simulink model "AdmittanceScanPRBS"  (R2025a)
settings: Solver=VariableStepAuto  StartTime=0.0  StopTime=Tsim  RelTol=1e-3
PreLoadFcn:
  | SimulationTime = 10;
  | AdmittanceScanParameters;
undefined symbols (not defined in the file): Array, Base, BatteryInverter, DiscIntNeverNeededParam, ee_sli_rtmsupport, feeder, fRT, frt, gcbh, GFLBatteryController, GFMBatteryController, gGFM, grid, Grid, line, loadpq, loadstep1, loadstep2, lvrt, LVRT, mGFM, Panel, pll, pmsm, PVController, PVInverter, PVTransformer, scan, time, Ts, VSMbase, windController, windTurbine
libraries: ee_lib x19, eeGeneralControl x17, nesl_utility x16, fl_lib x10, eeTransforms x9, simulink x8, slpidlib x2, batteryecm_lib x1, simulink_extras x1, eePowerMeasurement x1
(part 4 of 4)

== system AdmittanceScanPRBS/Renewable Plant/PV Plant/60 MWhr Battery Energy Storage/Variant Subsystem/Grid Forming VSM/GridFormingController/Power Control/ReactiveControl ==
  note: Vs-delV
  Qref : Inport
  Qmeas : Inport  Port=2
  Constant : Constant  Value=voltreference
  Constant2 : Constant  Value=0
  Gain : Gain  Gain=QVoltDroop
  Low-Pass Filter (Discrete or Continuous) : eeGeneralControl/Low-Pass Filter (Discrete or Continuous)  K=1  T=QVoltFilterTC  B=inf  A=-inf  init_option=Specify as parameter  x0=0  Ts=activePowerSampleTime
  Rate Transition : RateTransition
  Rate Transition1 : RateTransition
  Saturation1 : Saturate  UpperLimit=(dcBusVoltage/2)/(sqrt(2/3)*girdLineVoltage)  LowerLimit=-(dcBusVoltage/2)/(sqrt(2/3)*girdLineVoltage)
  Sum : Sum  Inputs=|+-
  Sum1 : Sum  Inputs=|++
  Vmd : Outport
  Vmq : Outport  Port=2
  wires:
  Sum/1 -> Gain/1
  Qmeas/1 -> Low-Pass Filter (Discrete or Continuous)/1
  Low-Pass Filter (Discrete or Continuous)/1 -> Rate Transition1/1
  Gain/1 -> Sum1/1
  Sum1/1 -> Saturation1/1  "Q"
  Constant/1 -> Sum1/2
  Constant2/1 -> Vmq/1
  Qref/1 -> Rate Transition/1
  Saturation1/1 -> Vmd/1
  Rate Transition/1 -> Sum/1
  Rate Transition1/1 -> Sum/2

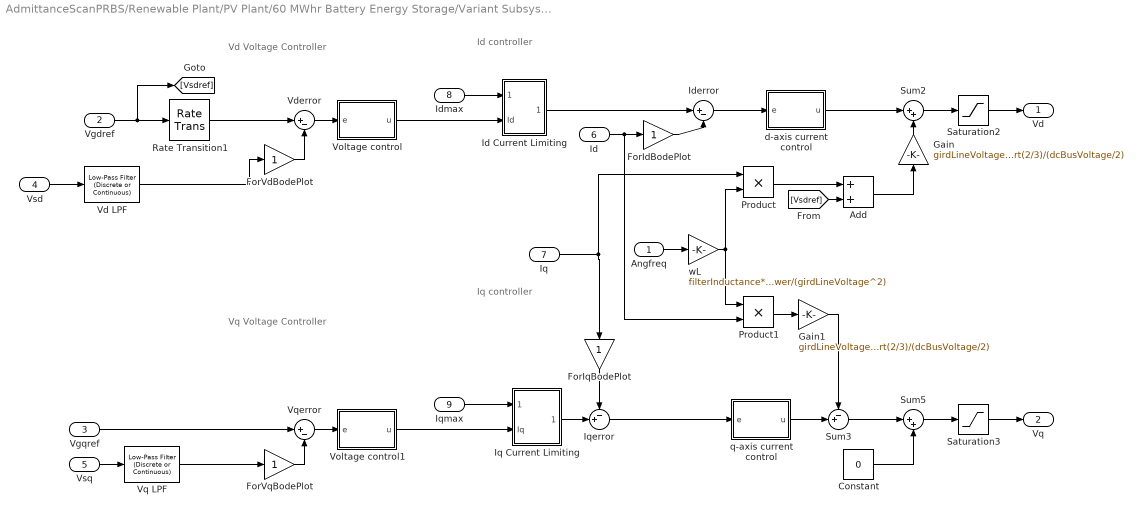
== system AdmittanceScanPRBS/Renewable Plant/PV Plant/60 MWhr Battery Energy Storage/Variant Subsystem/Grid Forming VSM/GridFormingController/VoltageCurrentControl/Controller ==
  note: Id controller
  note: Vd Voltage Controller
  note: Iq controller
  note: Vq Voltage Controller
  Angfreq : Inport
  Vgdref : Inport  Port=2
  Vgqref : Inport  Port=3
  Vsd : Inport  Port=4
  Vsq : Inport  Port=5
  Id : Inport  Port=6
  Iq : Inport  Port=7
  Idmax : Inport  Port=8
  Iqmax : Inport  Port=9
  Add : Sum
  Constant : Constant  Value=0  SampleTime=currentControlTs
  ForIdBodePlot : Gain
  ForIqBodePlot : Gain
  ForVdBodePlot : Gain
  ForVqBodePlot : Gain
  Gain : Gain  Gain=girdLineVoltage*sqrt(2/3)/(dcBusVoltage/2)
  Gain1 : Gain  Gain=girdLineVoltage*sqrt(2/3)/(dcBusVoltage/2)
  Id Current Limiting : Subsystem
  Iderror : Sum  Inputs=|+-
  Iq Current Limiting : Subsystem
  Iqerror : Sum  Inputs=-+|
  Product : Product
  Product1 : Product
  Rate Transition1 : RateTransition
  Saturation2 : Saturate  UpperLimit=4  LowerLimit=-3
  Saturation3 : Saturate  UpperLimit=3  LowerLimit=-3
  Sum2 : Sum  Inputs=|++
  Sum3 : Sum  Inputs=-+|
  Sum5 : Sum  Inputs=|++
  Vd LPF : eeGeneralControl/Low-Pass Filter (Discrete or Continuous)  K=1  T=vdvqLPFTimeConst  B=inf  A=-inf  init_option=Specify as parameter  x0=0  Ts=voltControlTs
  Vderror : Sum  Inputs=|+-
  Voltage control : Subsystem
  Voltage control1 : Subsystem
  Vq LPF : eeGeneralControl/Low-Pass Filter (Discrete or Continuous)  K=1  T=vdvqLPFTimeConst  B=inf  A=-inf  init_option=Inherited from block input  x0=0  Ts=voltControlTs
  Vqerror : Sum  Inputs=|+-
  d-axis current control : Subsystem
  q-axis current control : Subsystem
  wL : Gain  Gain=filterInductance*power/(girdLineVoltage^2)
  Vd : Outport  VectorParamsAs1DForOutWhenUnconnected=off
  Vq : Outport  Port=2  VectorParamsAs1DForOutWhenUnconnected=off
  wires:
  Iqerror/1 -> q-axis current control/1(e)
  wL/1 -> Product1/1, Product/2
  Iq/1 -> ForIqBodePlot/1, Product/1
  Angfreq/1 -> wL/1
  Constant/1 -> Sum5/2
  Iderror/1 -> d-axis current control/1(e)
  Saturation3/1 -> Vq/1
  Saturation2/1 -> Vd/1
  Product1/1 -> Gain1/1
  Product/1 -> Add/1
  d-axis current control/1(u) -> Sum2/1
  Sum2/1 -> Saturation2/1
  q-axis current control/1(u) -> Sum3/2
  Sum3/1 -> Sum5/1
  Sum5/1 -> Saturation3/1
  Vsq/1 -> Vq LPF/1
  Id/1 -> Product1/2, ForIdBodePlot/1
  Vderror/1 -> Voltage control/1(e)
  Iqmax/1 -> Iq Current Limiting/1(Imax)
  Vgqref/1 -> Vqerror/1
  Vqerror/1 -> Voltage control1/1(e)
  Gain1/1 -> Sum3/1
  [Vsdref] -> Add/2
  Add/1 -> Gain/1
  Gain/1 -> Sum2/2
  Voltage control/1(u) -> Id Current Limiting/2(Id)
  Idmax/1 -> Id Current Limiting/1(Imax)
  Iq Current Limiting/1(Iqref) -> Iqerror/2
  Voltage control1/1(u) -> Iq Current Limiting/2(Iq)
  Vsd/1 -> Vd LPF/1
  ForVdBodePlot/1 -> Vderror/2
  ForVqBodePlot/1 -> Vqerror/2
  ForIdBodePlot/1 -> Iderror/2
  ForIqBodePlot/1 -> Iqerror/1
  Id Current Limiting/1(Idref) -> Iderror/1
  Vq LPF/1 -> ForVqBodePlot/1
  Vgdref/1 -> Rate Transition1/1, [Vsdref]
  Vd LPF/1 -> ForVdBodePlot/1
  Rate Transition1/1 -> Vderror/1

== system AdmittanceScanPRBS/Renewable Plant/PV Plant/60 MWhr Battery Energy Storage/Variant Subsystem/Grid Forming VSM/GridFormingController/VoltageCurrentControl/Modulation Signal ==
  Vd : Inport
  Vq : Inport  Port=2
  Angle : Inport  Port=3
  Constant : Constant  Value=0
  Inverse Park Transform : eeTransforms/Inverse Park Transform  AxisAlignment=D-axis  PowerInvariant=off
  Mux1 : Mux  Inputs=3
  Saturation2 : Saturate  UpperLimit=1  LowerLimit=-1
  mabc : Outport  VectorParamsAs1DForOutWhenUnconnected=off
  wires:
  Inverse Park Transform/1 -> Saturation2/1
  Mux1/1 -> Inverse Park Transform/1
  Angle/1 -> Inverse Park Transform/2
  Saturation2/1 -> mabc/1
  Constant/1 -> Mux1/3
  Vd/1 -> Mux1/1
  Vq/1 -> Mux1/2

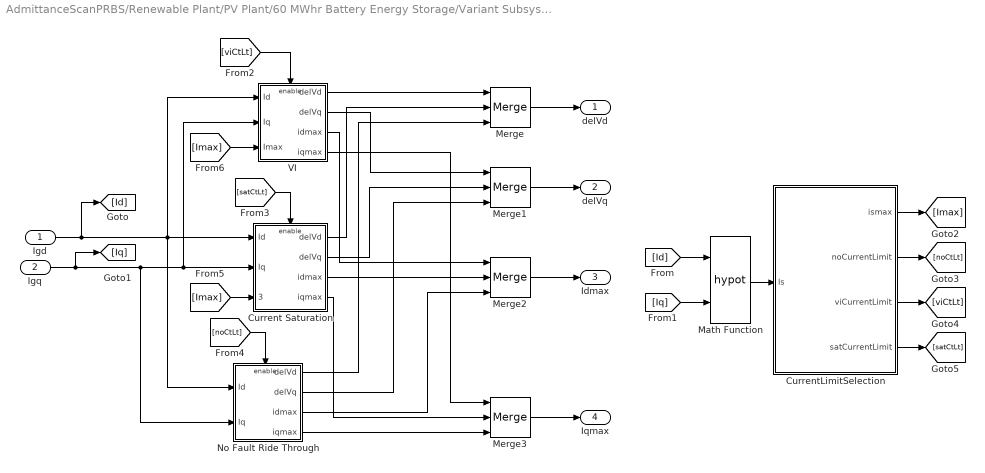
== system AdmittanceScanPRBS/Renewable Plant/PV Plant/60 MWhr Battery Energy Storage/Variant Subsystem/Grid Forming VSM/GridFormingController/Current Limiting/CurrentLimitingMethod/currentLimitAndVirtual ==
  Igd : Inport
  Igq : Inport  Port=2
  Current Saturation : Subsystem
  CurrentLimitSelection : Stateflow chart  TreatAsAtomicUnit=on
  Math Function : Math  Operator=hypot
  Merge{,1..3} (4 alike) : Merge  Inputs=3
  No Fault Ride Through : Subsystem
  VI : Subsystem
  delVd : Outport
  delVq : Outport  Port=2
  Idmax : Outport  Port=3
  Iqmax : Outport  Port=4
  wires:
  Merge2/1 -> Idmax/1
  Igq/1 -> Current Saturation/2(Iq), VI/2(Iq), No Fault Ride Through/2(Iq), [Iq]
  Merge1/1 -> delVq/1
  Igd/1 -> VI/1(Id), Current Saturation/1(Id), No Fault Ride Through/1(Id), [Id]
  No Fault Ride Through/1(delVd) -> Merge/3
  No Fault Ride Through/3(idmax) -> Merge2/3
  VI/1(delVd) -> Merge/1
  [Iq] -> Math Function/2
  [Id] -> Math Function/1
  Current Saturation/1(delVd) -> Merge/2
  Current Saturation/4(iqmax) -> Merge3/2
  Merge/1 -> delVd/1
  VI/2(delVq) -> Merge1/1
  Current Saturation/3(idmax) -> Merge2/2
  VI/4(iqmax) -> Merge3/1
  VI/3(idmax) -> Merge2/1
  No Fault Ride Through/4(iqmax) -> Merge3/3
  Current Saturation/2(delVq) -> Merge1/2
  Merge3/1 -> Iqmax/1
  No Fault Ride Through/2(delVq) -> Merge1/3
  Math Function/1 -> CurrentLimitSelection/1(Is)
  CurrentLimitSelection/1(ismax) -> [Imax]
  CurrentLimitSelection/2(noCurrentLimit) -> [noCtLt]
  CurrentLimitSelection/3(viCurrentLimit) -> [viCtLt]
  CurrentLimitSelection/4(satCurrentLimit) -> [satCtLt]
  [viCtLt] -> VI/Enable
  [satCtLt] -> Current Saturation/Enable
  [noCtLt] -> No Fault Ride Through/Enable
  [Imax] -> Current Saturation/3(Imaxsat)
  [Imax] -> VI/3(Imax)

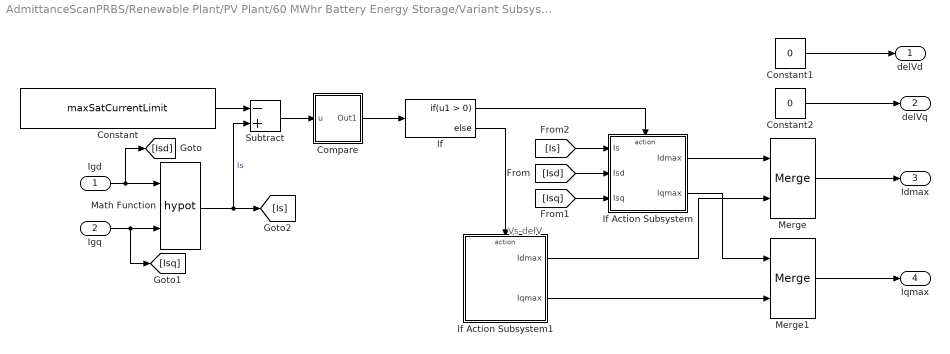
== system AdmittanceScanPRBS/Renewable Plant/PV Plant/60 MWhr Battery Energy Storage/Variant Subsystem/Grid Forming VSM/GridFormingController/Current Limiting/CurrentLimitingMethod/currentSaturation ==
  note: Vs-delV
  Igd : Inport
  Igq : Inport  Port=2
  Compare : Subsystem
  Constant : Constant  Value=maxSatCurrentLimit
  Constant1 : Constant  Value=0
  Constant2 : Constant  Value=0
  If : If
  If Action Subsystem : Subsystem  TreatAsAtomicUnit=on
  If Action Subsystem1 : Subsystem  TreatAsAtomicUnit=on
  Math Function : Math  Operator=hypot
  Merge : Merge
  Merge1 : Merge
  Subtract : Sum  Inputs=-+
  delVd : Outport
  delVq : Outport  Port=2
  Idmax : Outport  Port=3
  Iqmax : Outport  Port=4
  wires:
  Igd/1 -> [Isd], Math Function/1
  Igq/1 -> [Isq], Math Function/2
  Constant/1 -> Subtract/1
  Math Function/1 -> [Is], Subtract/2  "Is"
  If/1 -> If Action Subsystem/Action
  [Isd] -> If Action Subsystem/2(Isd)
  [Isq] -> If Action Subsystem/3(Isq)
  Subtract/1 -> Compare/1(u)
  Compare/1(Out1) -> If/1
  If/2 -> If Action Subsystem1/Action
  [Is] -> If Action Subsystem/1(Is)
  If Action Subsystem/1(Idmax) -> Merge/1
  If Action Subsystem1/1(Idmax) -> Merge/2
  If Action Subsystem/2(Iqmax) -> Merge1/1
  If Action Subsystem1/2(Iqmax) -> Merge1/2
  Constant2/1 -> delVq/1
  Constant1/1 -> delVd/1
  Merge/1 -> Idmax/1
  Merge1/1 -> Iqmax/1

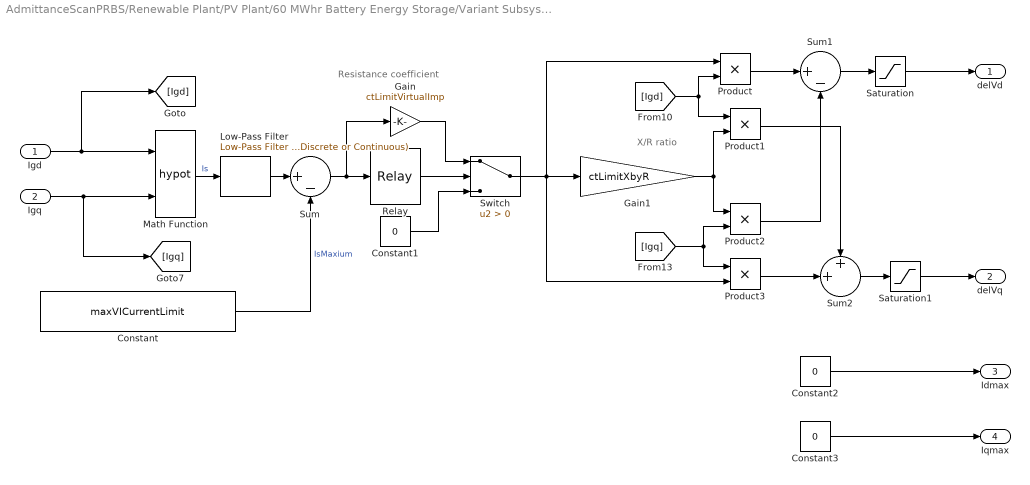
== system AdmittanceScanPRBS/Renewable Plant/PV Plant/60 MWhr Battery Energy Storage/Variant Subsystem/Grid Forming VSM/GridFormingController/Current Limiting/CurrentLimitingMethod/virtualImpedance ==
  note: X/R ratio
  note: Resistance coefficient
  Igd : Inport
  Igq : Inport  Port=2
  Constant : Constant  Value=maxVICurrentLimit
  Constant1 : Constant  Value=0
  Constant2 : Constant  Value=0
  Constant3 : Constant  Value=0
  Gain : Gain  Gain=ctLimitVirtualImp
  Gain1 : Gain  Gain=ctLimitXbyR
  Low-Pass Filter : eeGeneralControl/Low-Pass Filter (Discrete or Continuous)  K=1  T=currentVITimeConst  B=inf  A=-inf  init_option=Inherited from block input  x0=0  Ts=-1
  Math Function : Math  Operator=hypot
  Product{,1..3} (4 alike) : Product
  Relay : Relay  OnSwitchValue=0.01  OffSwitchValue=-0.05
  Saturation : Saturate  UpperLimit=1  LowerLimit=-1
  Saturation1 : Saturate  UpperLimit=1  LowerLimit=-1
  Sum : Sum  Inputs=|+-
  Sum1 : Sum  Inputs=|+-
  Sum2 : Sum  Inputs=++|
  Switch : Switch  Criteria=u2 > Threshold  SaturateOnIntegerOverflow=off  InputSameDT=off
  delVd : Outport
  delVq : Outport  Port=2
  Idmax : Outport  Port=3
  Iqmax : Outport  Port=4
  wires:
  Sum/1 -> Gain/1, Relay/1
  Igq/1 -> [Igq], Math Function/2
  Product1/1 -> Sum2/1
  Gain1/1 -> Product1/2, Product2/1
  Sum1/1 -> Saturation/1
  Product/1 -> Sum1/1
  Product2/1 -> Sum1/2
  Constant/1 -> Sum/2  "IsMaxium"
  Math Function/1 -> Low-Pass Filter/1  "Is"
  [Igq] -> Product3/1, Product2/2
  Switch/1 -> Gain1/1, Product3/2, Product/1
  [Igd] -> Product1/1, Product/2
  Constant2/1 -> Idmax/1
  Constant3/1 -> Iqmax/1
  Gain/1 -> Switch/1
  Constant1/1 -> Switch/3
  Igd/1 -> Math Function/1, [Igd]
  Saturation1/1 -> delVq/1
  Relay/1 -> Switch/2
  Saturation/1 -> delVd/1
  Low-Pass Filter/1 -> Sum/1
  Product3/1 -> Sum2/2
  Sum2/1 -> Saturation1/1

== system AdmittanceScanPRBS/Renewable Plant/PV Plant/60 MWhr Battery Energy Storage/Variant Subsystem/Grid Forming VSM/GridFormingController/Grid Voltage Reactive Power Support/Modifying Active Power Reference/Computing New Active Power Ref ==
  Iq : Inport
  Vd : Inport  Port=2
  Abs : Abs  SaturateOnIntegerOverflow=off
  Constant : Constant  Value=maxVICurrentLimit*0.96
  Constant1 : Constant  Value=0
  Product : Product
  Sqrt : Sqrt
  Square : Math  Operator=square
  Square1 : Math  Operator=square
  Subtract : Sum  Inputs=-+
  Switch : Switch  Criteria=u2 > Threshold  Threshold=1.15  SaturateOnIntegerOverflow=off  InputSameDT=off
  Pref : Outport
  wires:
  Constant/1 -> Square1/1
  Switch/1 -> Product/2
  Square/1 -> Subtract/1
  Square1/1 -> Subtract/2
  Vd/1 -> Product/1
  Sqrt/1 -> Abs/1
  Iq/1 -> Square/1
  Product/1 -> Pref/1
  Subtract/1 -> Switch/2, Sqrt/1
  Constant1/1 -> Switch/3
  Abs/1 -> Switch/1

== system AdmittanceScanPRBS/Renewable Plant/PV Plant/60 MWhr Battery Energy Storage/Variant Subsystem/Grid Forming VSM/GridFormingController/Grid Voltage Reactive Power Support/Modifying Reactive Power Reference/Changing the Power Reference ==
  Vs : Inport
  Vd : Inport  Port=2
  Pref : Inport  Port=3
  Qref : Inport  Port=4
  Enable : EnablePort
  ActivePowerReference : Subsystem
  Constant1 : Constant  Value=voltreference*0.96
  Estimate Id for Given Iq : Subsystem
  EstimateIqForReactivePower : Subsystem
  Max : MinMax  Function=max  Inputs=2
  Rate Transition1 : RateTransition
  ReactivePowerReference : Subsystem
  Prefv : Outport
  Qrefv : Outport  Port=2
  wires:
  EstimateIqForReactivePower/1(Iq) -> Estimate Id for Given Iq/1(Iq), ReactivePowerReference/2(Iq)
  Constant1/1 -> EstimateIqForReactivePower/1(Vmin)
  Vs/1 -> Rate Transition1/1
  Estimate Id for Given Iq/1(Id) -> ActivePowerReference/1(Id)
  Pref/1 -> ActivePowerReference/3(Pref)
  ReactivePowerReference/1(QrefNew) -> Max/1
  Qref/1 -> Max/2
  Vd/1 -> EstimateIqForReactivePower/2(Vd)
  Max/1 -> Qrefv/1
  ActivePowerReference/1(PrefNew) -> Prefv/1
  Rate Transition1/1 -> EstimateIqForReactivePower/3(Vs), ReactivePowerReference/1(Vd), ActivePowerReference/2(Vd)

== system AdmittanceScanPRBS/Renewable Plant/PV Plant/60 MWhr Battery Energy Storage/Variant Subsystem/Grid Forming VSM/GridFormingController/Grid Voltage Reactive Power Support/Modifying Reactive Power Reference/Hysteresis ==
  Vs : Inport
  AND : Logic  IconShape=distinctive  AllPortsSameDT=off  OutDataTypeStr=boolean
  Compare To Constant : simulink/Logic and Bit Operations/Compare To Constant  relop=<  const=0.9  OutDataTypeStr=boolean
  Compare To Constant1 : simulink/Logic and Bit Operations/Compare To Constant  relop=<  const=0.95  OutDataTypeStr=boolean
  D Latch : simulink_extras/Flip Flops/D Latch
  OR : Logic  Operator=OR  IconShape=distinctive  AllPortsSameDT=off  OutDataTypeStr=boolean
  Terminator : Terminator
  LVFlag : Outport
  wires:
  Compare To Constant1/1 -> AND/1
  D Latch/1 -> AND/2
  AND/1 -> OR/1
  OR/1 -> LVFlag/1
  D Latch/2 -> Terminator/1
  Compare To Constant/1 -> D Latch/1, D Latch/2, OR/2
  Vs/1 -> Compare To Constant1/1, Compare To Constant/1

== system AdmittanceScanPRBS/Renewable Plant/PV Plant/60 MWhr Battery Energy Storage/Variant Subsystem/Grid Forming VSM/GridFormingController/Grid Voltage Reactive Power Support/Modifying Reactive Power Reference/Not Altering the Power Reference ==
  Pref : Inport
  Qref : Inport  Port=2
  Enable : EnablePort
  Prefv : Outport
  Qrefv : Outport  Port=2
  wires:
  Pref/1 -> Prefv/1
  Qref/1 -> Qrefv/1

== system AdmittanceScanPRBS/Renewable Plant/PV Plant/60 MWhr Battery Energy Storage/Variant Subsystem/Grid Forming VSM/GridFormingController/Measurement/Frequency Measurement/Frequency Measurement ==
  abc : Inport
  Constant : Constant
  Discrete-Time Integrator : DiscreteIntegrator  SampleTime=sampleTime  LimitOutput=on  ICPrevOutput=DiscIntNeverNeededParam  ICPrevScaledInput=DiscIntNeverNeededParam
  If : If  IfExpression=u1 > 0.9
  If Action Subsystem : Subsystem  TreatAsAtomicUnit=on
  If Action Subsystem1 : Subsystem  TreatAsAtomicUnit=on
  Merge : Merge
  Postive Sequence : Subsystem
  Freq : Outport
  wires:
  If/1 -> If Action Subsystem/Action
  If/2 -> If Action Subsystem1/Action
  Discrete-Time Integrator/1 -> If Action Subsystem/2(Time), If/1
  abc/1 -> Postive Sequence/1(abc)
  Constant/1 -> Discrete-Time Integrator/1
  If Action Subsystem/1(Freq) -> Merge/1
  If Action Subsystem1/1(Out1) -> Merge/2
  Merge/1 -> Freq/1
  Postive Sequence/1(posSeq) -> If Action Subsystem/1(V)

== system AdmittanceScanPRBS/Renewable Plant/PV Plant/60 MWhr Battery Energy Storage/Variant Subsystem/Grid Forming VSM/GridFormingController/Measurement/abc2dq/Supply Current to dq ==
  abc : Inport
  Angle : Inport  Port=2
  Demux : Demux  Outputs=3
  Park Transform : eeTransforms/Park Transform  AxisAlignment=D-axis  PowerInvariant=off
  Terminator : Terminator
  Igd : Outport  VectorParamsAs1DForOutWhenUnconnected=off
  Igq : Outport  Port=2  VectorParamsAs1DForOutWhenUnconnected=off
  wires:
  Demux/3 -> Terminator/1
  Park Transform/1 -> Demux/1
  Demux/2 -> Igq/1
  Demux/1 -> Igd/1
  abc/1 -> Park Transform/1
  Angle/1 -> Park Transform/2

== system AdmittanceScanPRBS/Renewable Plant/PV Plant/60 MWhr Battery Energy Storage/Variant Subsystem/Grid Forming VSM/GridFormingController/Measurement/abc2dq/Supply Voltage  to dq ==
  Angle : Inport
  abc : Inport  Port=2
  Demux : Demux  Outputs=3
  Park Transform : eeTransforms/Park Transform  AxisAlignment=D-axis  PowerInvariant=off
  Terminator : Terminator
  Vgd : Outport  VectorParamsAs1DForOutWhenUnconnected=off
  Vgq : Outport  Port=2  VectorParamsAs1DForOutWhenUnconnected=off
  wires:
  Demux/3 -> Terminator/1
  Park Transform/1 -> Demux/1
  Demux/2 -> Vgq/1
  Demux/1 -> Vgd/1
  abc/1 -> Park Transform/1
  Angle/1 -> Park Transform/2

== system AdmittanceScanPRBS/Renewable Plant/PV Plant/60 MWhr Battery Energy Storage/Variant Subsystem/Grid Forming VSM/GridFormingController/Power Control/ActivePowerControl/droopControl ==
  Pref : Inport
  Pmeas : Inport  Port=2
  fgrid : Inport  Port=3
  Add : Sum  Inputs=+-
  Constant : Constant
  Constant5 : Constant  Value=pi/2
  Gain : Gain  Gain=powerFreq*2*pi
  Integrator with Wrapped State (Discrete or Continuous) : eeGeneralControl/Integrator with Wrapped State (Discrete or Continuous)  LabelModeActiveChoice=Discrete  WrappedStateUpperValue=2*pi  WrappedStateLowerValue=0  x0=0  Ts=activePowerSampleTime
      settings: LibrarySourceBlock=|
      | ee_sl_lib/General Control/Integrator with
      | Wrapped State
      | (Discrete or Continuous)
  Lead-Lag (Discrete or Continuous) : eeGeneralControl/Lead-Lag (Discrete or Continuous)  T1=droopT1  T2=droopT2  B=inf  A=-inf  init_option=Inherited from block input  x0=0  Ts=activePowerSampleTime
      settings: LibrarySourceBlock=|
      | ee_sl_lib/General Control/Lead-Lag
      | (Discrete or Continuous)
  Low-Pass Filter (Discrete or Continuous) : eeGeneralControl/Low-Pass Filter (Discrete or Continuous)  K=1  T=droopTC  B=inf  A=-inf  init_option=Specify as parameter  x0=0  Ts=activePowerSampleTime
  Sum : Sum  Inputs=|-+
  Sum1 : Sum  Inputs=|-+
  Terminator : Terminator
  mp : Gain  Gain=droopSlope
  Theta : Outport
  w : Outport  Port=2
  wires:
  Low-Pass Filter (Discrete or Continuous)/1 -> Sum1/1
  mp/1 -> Low-Pass Filter (Discrete or Continuous)/1
  Sum/1 -> mp/1
  Pmeas/1 -> Lead-Lag (Discrete or Continuous)/1
  Add/1 -> Theta/1
  Constant5/1 -> Add/2
  Pref/1 -> Sum/1
  Gain/1 -> Integrator with Wrapped State (Discrete or Continuous)/1, w/1
  Lead-Lag (Discrete or Continuous)/1 -> Sum/2
  Integrator with Wrapped State (Discrete or Continuous)/1 -> Add/1
  Constant/1 -> Sum1/2
  Sum1/1 -> Gain/1
  fgrid/1 -> Terminator/1

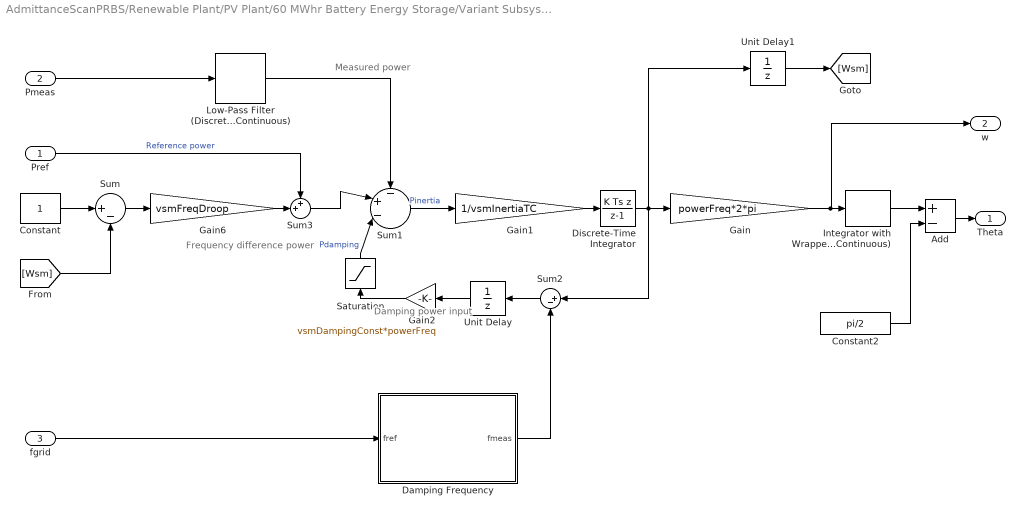
== system AdmittanceScanPRBS/Renewable Plant/PV Plant/60 MWhr Battery Energy Storage/Variant Subsystem/Grid Forming VSM/GridFormingController/Power Control/ActivePowerControl/vsmControl ==
  note: Measured power
  note: Frequency difference power
  note: Damping power input
  Pref : Inport
  Pmeas : Inport  Port=2
  fgrid : Inport  Port=3
  Add : Sum  Inputs=+-
  Constant : Constant
  Constant2 : Constant  Value=pi/2
  Damping Frequency : Subsystem  Variant=on  VariantControlMode=label  VariantControl=Choice  LabelModeActiveChoice=freqMeas
  Discrete-Time Integrator : DiscreteIntegrator  IntegratorMethod=Integration: Backward Euler  InitialCondition=1  SampleTime=activePowerSampleTime  LimitOutput=on  UpperSaturationLimit=1.1  LowerSaturationLimit=0.9  ICPrevOutput=DiscIntNeverNeededParam  ICPrevScaledInput=DiscIntNeverNeededParam
  Gain : Gain  Gain=powerFreq*2*pi
  Gain1 : Gain  Gain=1/vsmInertiaTC
  Gain2 : Gain  Gain=vsmDampingConst*powerFreq
  Gain6 : Gain  Gain=vsmFreqDroop
  Integrator with Wrapped State (Discrete or Continuous) : eeGeneralControl/Integrator with Wrapped State (Discrete or Continuous)  LabelModeActiveChoice=Discrete  WrappedStateUpperValue=2*pi  WrappedStateLowerValue=0  x0=0  Ts=activePowerSampleTime
      settings: LibrarySourceBlock=|
      | ee_sl_lib/General Control/Integrator with
      | Wrapped State
      | (Discrete or Continuous)
  Low-Pass Filter (Discrete or Continuous) : eeGeneralControl/Low-Pass Filter (Discrete or Continuous)  K=1  T=vsmPmeasFilterTC  B=inf  A=-inf  init_option=Specify as parameter  x0=0  Ts=activePowerSampleTime
  Saturation : Saturate  UpperLimit=dampingPowerMaxLimit  LowerLimit=dampingPowerMinLimit
  Sum : Sum  Inputs=|+-
  Sum1 : Sum  Inputs=-+-|
  Sum2 : Sum  Inputs=|+-
  Sum3 : Sum  Inputs=++|
  Unit Delay : UnitDelay  SampleTime=-1  HasFrameUpgradeWarning=on
  Unit Delay1 : UnitDelay  SampleTime=-1  HasFrameUpgradeWarning=on
  Theta : Outport
  w : Outport  Port=2
  wires:
  Integrator with Wrapped State (Discrete or Continuous)/1 -> Add/1
  Sum1/1 -> Gain1/1  "Pinertia"
  Sum/1 -> Gain6/1
  Constant2/1 -> Add/2
  Add/1 -> Theta/1
  Pmeas/1 -> Low-Pass Filter (Discrete or Continuous)/1
  Discrete-Time Integrator/1 -> Gain/1, Unit Delay1/1, Sum2/1
  [Wsm] -> Sum/2
  Low-Pass Filter (Discrete or Continuous)/1 -> Sum1/1
  Pref/1 -> Sum3/1  "Reference power"
  Gain2/1 -> Saturation/1
  Sum3/1 -> Sum1/2
  Sum2/1 -> Unit Delay/1
  Gain1/1 -> Discrete-Time Integrator/1
  Gain/1 -> Integrator with Wrapped State (Discrete or Continuous)/1, w/1
  Unit Delay/1 -> Gain2/1
  Constant/1 -> Sum/1
  Unit Delay1/1 -> [Wsm]
  Saturation/1 -> Sum1/3  "Pdamping"
  Gain6/1 -> Sum3/2
  fgrid/1 -> Damping Frequency/1(fref)
  Damping Frequency/1(fmeas) -> Sum2/2

== system AdmittanceScanPRBS/Renewable Plant/PV Plant/60 MWhr Battery Energy Storage/Variant Subsystem/Grid Forming VSM/GridFormingController/VoltageCurrentControl/Controller/Id Current Limiting ==
  Imax : Inport
  Id : Inport  Port=2
  Abs : Abs  SaturateOnIntegerOverflow=off
  Rate Transition : RateTransition
  Switch : Switch  Criteria=u2 > Threshold  SaturateOnIntegerOverflow=off  InputSameDT=off
  Idref : Outport
  wires:
  Id/1 -> Rate Transition/1
  Abs/1 -> Switch/2
  Imax/1 -> Abs/1, Switch/1
  Switch/1 -> Idref/1
  Rate Transition/1 -> Switch/3

== system AdmittanceScanPRBS/Renewable Plant/PV Plant/60 MWhr Battery Energy Storage/Variant Subsystem/Grid Forming VSM/GridFormingController/VoltageCurrentControl/Controller/Iq Current Limiting ==
  Imax : Inport
  Iq : Inport  Port=2
  Abs : Abs  SaturateOnIntegerOverflow=off
  Switch : Switch  Criteria=u2 > Threshold  SaturateOnIntegerOverflow=off  InputSameDT=off
  Iqref : Outport
  wires:
  Iq/1 -> Switch/3
  Abs/1 -> Switch/2
  Imax/1 -> Abs/1, Switch/1
  Switch/1 -> Iqref/1

== system AdmittanceScanPRBS/Renewable Plant/PV Plant/60 MWhr Battery Energy Storage/Variant Subsystem/Grid Forming VSM/GridFormingController/VoltageCurrentControl/Controller/Voltage control ==
  e : Inport
  Discrete-Time Integrator : DiscreteIntegrator  IntegratorMethod=Integration: Backward Euler  SampleTime=voltControlTs  LimitOutput=on  UpperSaturationLimit=VdMaxCt  LowerSaturationLimit=VdMinCt  ICPrevOutput=DiscIntNeverNeededParam  ICPrevScaledInput=DiscIntNeverNeededParam
  Ki : Gain  Gain=VdIGain
  Kp : Gain  Gain=vdPGain
  Limit : Saturate  UpperLimit=VdMaxCt  LowerLimit=VdMinCt
  Sum7 : Sum  Inputs=|++
  u : Outport  VectorParamsAs1DForOutWhenUnconnected=off
  wires:
  Discrete-Time Integrator/1 -> Sum7/2
  Kp/1 -> Sum7/1
  Limit/1 -> u/1
  Ki/1 -> Discrete-Time Integrator/1
  Sum7/1 -> Limit/1
  e/1 -> Kp/1, Ki/1

== system AdmittanceScanPRBS/Renewable Plant/PV Plant/60 MWhr Battery Energy Storage/Variant Subsystem/Grid Forming VSM/GridFormingController/VoltageCurrentControl/Controller/Voltage control1 ==
  e : Inport
  Discrete-Time Integrator : DiscreteIntegrator  IntegratorMethod=Integration: Backward Euler  SampleTime=voltControlTs  LimitOutput=on  UpperSaturationLimit=VqMaxCt  LowerSaturationLimit=VqMinCt  ICPrevOutput=DiscIntNeverNeededParam  ICPrevScaledInput=DiscIntNeverNeededParam
  Ki : Gain  Gain=VqIGain
  Kp : Gain  Gain=VqPGain
  Limit : Saturate  UpperLimit=VqMaxCt  LowerLimit=VqMinCt
  Sum7 : Sum  Inputs=|++
  u : Outport  VectorParamsAs1DForOutWhenUnconnected=off
  wires:
  Discrete-Time Integrator/1 -> Sum7/2
  Sum7/1 -> Limit/1
  e/1 -> Ki/1, Kp/1
  Kp/1 -> Sum7/1
  Ki/1 -> Discrete-Time Integrator/1
  Limit/1 -> u/1

== system AdmittanceScanPRBS/Renewable Plant/PV Plant/60 MWhr Battery Energy Storage/Variant Subsystem/Grid Forming VSM/GridFormingController/VoltageCurrentControl/Controller/d-axis current control ==
  e : Inport
  Discrete-Time Integrator : DiscreteIntegrator  IntegratorMethod=Integration: Backward Euler  SampleTime=currentControlTs  LimitOutput=on  UpperSaturationLimit=4  LowerSaturationLimit=-4  ICPrevOutput=DiscIntNeverNeededParam  ICPrevScaledInput=DiscIntNeverNeededParam
  Ki : Gain  Gain=IdIGain
  Kp : Gain  Gain=IdPGain
  Limit : Saturate  UpperLimit=4  LowerLimit=-4
  Sum7 : Sum  Inputs=|++
  u : Outport  VectorParamsAs1DForOutWhenUnconnected=off
  wires:
  Discrete-Time Integrator/1 -> Sum7/2
  Sum7/1 -> Limit/1
  e/1 -> Ki/1, Kp/1
  Kp/1 -> Sum7/1
  Limit/1 -> u/1
  Ki/1 -> Discrete-Time Integrator/1

== system AdmittanceScanPRBS/Renewable Plant/PV Plant/60 MWhr Battery Energy Storage/Variant Subsystem/Grid Forming VSM/GridFormingController/VoltageCurrentControl/Controller/q-axis current control ==
  e : Inport
  Discrete-Time Integrator : DiscreteIntegrator  IntegratorMethod=Integration: Backward Euler  SampleTime=currentControlTs  LimitOutput=on  UpperSaturationLimit=3  LowerSaturationLimit=-3  ICPrevOutput=DiscIntNeverNeededParam  ICPrevScaledInput=DiscIntNeverNeededParam
  Ki : Gain  Gain=IqIGain
  Kp : Gain  Gain=IqPGain
  Limit : Saturate  UpperLimit=3  LowerLimit=-3
  Sum7 : Sum  Inputs=|++
  u : Outport  VectorParamsAs1DForOutWhenUnconnected=off
  wires:
  Ki/1 -> Discrete-Time Integrator/1
  Kp/1 -> Sum7/1
  e/1 -> Kp/1, Ki/1
  Sum7/1 -> Limit/1
  Limit/1 -> u/1
  Discrete-Time Integrator/1 -> Sum7/2

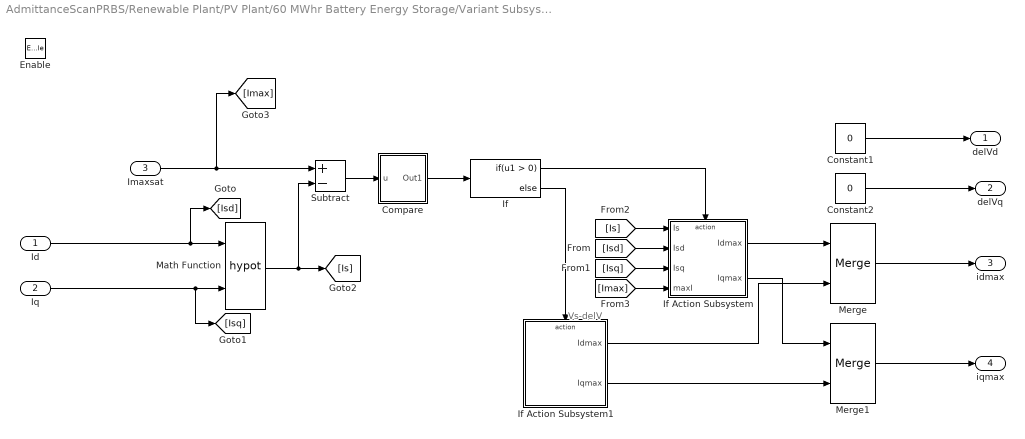
== system AdmittanceScanPRBS/Renewable Plant/PV Plant/60 MWhr Battery Energy Storage/Variant Subsystem/Grid Forming VSM/GridFormingController/Current Limiting/CurrentLimitingMethod/currentLimitAndVirtual/Current Saturation ==
  note: Vs-delV
  Id : Inport
  Iq : Inport  Port=2
  Imaxsat : Inport  Port=3
  Enable : EnablePort
  Compare : Subsystem
  Constant1 : Constant  Value=0
  Constant2 : Constant  Value=0
  If : If
  If Action Subsystem : Subsystem  TreatAsAtomicUnit=on
  If Action Subsystem1 : Subsystem  TreatAsAtomicUnit=on
  Math Function : Math  Operator=hypot
  Merge : Merge
  Merge1 : Merge
  Subtract : Sum  Inputs=+-
  delVd : Outport
  delVq : Outport  Port=2
  idmax : Outport  Port=3
  iqmax : Outport  Port=4
  wires:
  Iq/1 -> [Isq], Math Function/2
  If/1 -> If Action Subsystem/Action
  If Action Subsystem1/1(Idmax) -> Merge/2
  Constant2/1 -> delVq/1
  Math Function/1 -> [Is], Subtract/2
  If/2 -> If Action Subsystem1/Action
  If Action Subsystem/2(Iqmax) -> Merge1/1
  Subtract/1 -> Compare/1(u)
  Compare/1(Out1) -> If/1
  If Action Subsystem/1(Idmax) -> Merge/1
  [Is] -> If Action Subsystem/1(Is)
  Id/1 -> [Isd], Math Function/1
  If Action Subsystem1/2(Iqmax) -> Merge1/2
  Merge/1 -> idmax/1
  [Isd] -> If Action Subsystem/2(Isd)
  Constant1/1 -> delVd/1
  [Isq] -> If Action Subsystem/3(Isq)
  Merge1/1 -> iqmax/1
  Imaxsat/1 -> [Imax], Subtract/1
  [Imax] -> If Action Subsystem/4(maxI)

== system AdmittanceScanPRBS/Renewable Plant/PV Plant/60 MWhr Battery Energy Storage/Variant Subsystem/Grid Forming VSM/GridFormingController/Current Limiting/CurrentLimitingMethod/currentLimitAndVirtual/No Fault Ride Through ==
  Id : Inport
  Iq : Inport  Port=2
  Enable : EnablePort
  Constant{1..4} (4 alike) : Constant  Value=0
  Terminator : Terminator
  Terminator1 : Terminator
  delVd : Outport
  delVq : Outport  Port=2
  idmax : Outport  Port=3
  iqmax : Outport  Port=4
  wires:
  Constant3/1 -> iqmax/1
  Constant2/1 -> idmax/1
  Constant1/1 -> delVd/1
  Constant4/1 -> delVq/1
  Id/1 -> Terminator/1
  Iq/1 -> Terminator1/1

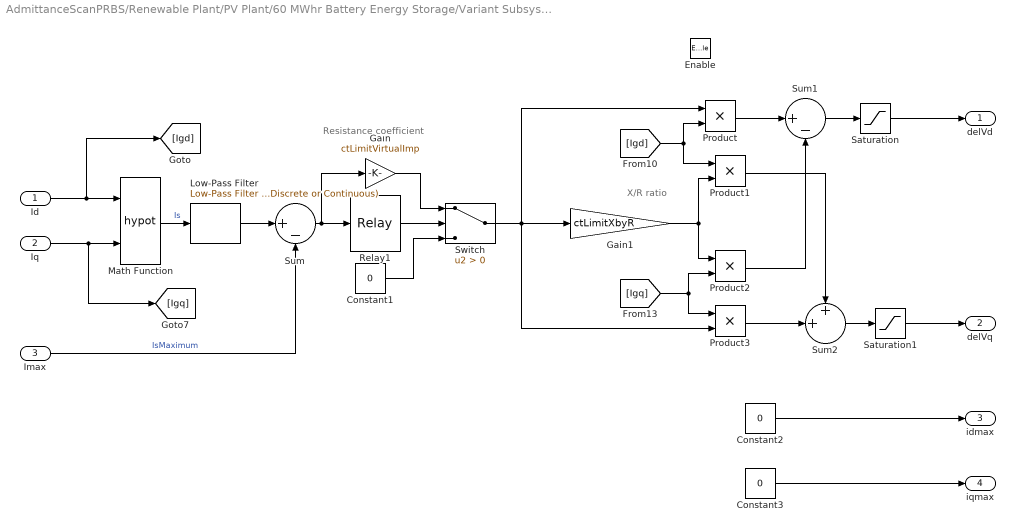
== system AdmittanceScanPRBS/Renewable Plant/PV Plant/60 MWhr Battery Energy Storage/Variant Subsystem/Grid Forming VSM/GridFormingController/Current Limiting/CurrentLimitingMethod/currentLimitAndVirtual/VI ==
  note: Resistance coefficient
  note: X/R ratio
  Id : Inport
  Iq : Inport  Port=2
  Imax : Inport  Port=3
  Enable : EnablePort
  Constant1 : Constant  Value=0
  Constant2 : Constant  Value=0
  Constant3 : Constant  Value=0
  Gain : Gain  Gain=ctLimitVirtualImp
  Gain1 : Gain  Gain=ctLimitXbyR
  Low-Pass Filter : eeGeneralControl/Low-Pass Filter (Discrete or Continuous)  K=1  T=currentVITimeConst  B=inf  A=-inf  init_option=Inherited from block input  x0=0  Ts=-1
  Math Function : Math  Operator=hypot
  Product{,1..3} (4 alike) : Product
  Relay1 : Relay  OnSwitchValue=0.01  OffSwitchValue=-0.1
  Saturation : Saturate  UpperLimit=1  LowerLimit=-1
  Saturation1 : Saturate  UpperLimit=1  LowerLimit=-1
  Sum : Sum  Inputs=|+-
  Sum1 : Sum  Inputs=|+-
  Sum2 : Sum  Inputs=++|
  Switch : Switch  Criteria=u2 > Threshold  SaturateOnIntegerOverflow=off  InputSameDT=off
  delVd : Outport
  delVq : Outport  Port=2
  idmax : Outport  Port=3
  iqmax : Outport  Port=4
  wires:
  Gain1/1 -> Product1/2, Product2/1
  Product3/1 -> Sum2/2
  Id/1 -> Math Function/1, [Igd]
  Sum2/1 -> Saturation1/1
  Sum/1 -> Gain/1, Relay1/1
  Sum1/1 -> Saturation/1
  Product/1 -> Sum1/1
  [Igq] -> Product3/1, Product2/2
  Iq/1 -> [Igq], Math Function/2
  Math Function/1 -> Low-Pass Filter/1  "Is"
  Switch/1 -> Product3/2, Product/1, Gain1/1
  [Igd] -> Product1/1, Product/2
  Saturation1/1 -> delVq/1
  Product1/1 -> Sum2/1
  Product2/1 -> Sum1/2
  Gain/1 -> Switch/1
  Constant1/1 -> Switch/3
  Saturation/1 -> delVd/1
  Constant3/1 -> iqmax/1
  Constant2/1 -> idmax/1
  Relay1/1 -> Switch/2
  Low-Pass Filter/1 -> Sum/1
  Imax/1 -> Sum/2  "IsMaximum"

== system AdmittanceScanPRBS/Renewable Plant/PV Plant/60 MWhr Battery Energy Storage/Variant Subsystem/Grid Forming VSM/GridFormingController/Current Limiting/CurrentLimitingMethod/currentSaturation/Compare ==
  u : Inport
  AND : Logic  IconShape=distinctive  AllPortsSameDT=off  OutDataTypeStr=boolean
  Compare To Constant : simulink/Logic and Bit Operations/Compare To Constant  relop=>  const=ctLimitDelayTime  OutDataTypeStr=boolean
  Data Type Conversion : DataTypeConversion  SaturateOnIntegerOverflow=off  RndMeth=Floor
  Data Type Conversion1 : DataTypeConversion  SaturateOnIntegerOverflow=off  RndMeth=Floor
  Discrete-Time Integrator : DiscreteIntegrator  IntegratorMethod=Integration: Backward Euler  ExternalReset=falling  SampleTime=currentControlTs  LimitOutput=on  UpperSaturationLimit=ctLimitDelayTime*2  LowerSaturationLimit=0  ICPrevOutput=DiscIntNeverNeededParam  ICPrevScaledInput=DiscIntNeverNeededParam
  Relay : Relay  OnSwitchValue=0.005*maxSatCurrentLimit  OffSwitchValue=-1*0.02*maxSatCurrentLimit
  Out1 : Outport
  wires:
  AND/1 -> Data Type Conversion/1
  Relay/1 -> Data Type Conversion1/1
  u/1 -> Relay/1
  Discrete-Time Integrator/1 -> Compare To Constant/1
  Data Type Conversion/1 -> Out1/1
  Data Type Conversion1/1 -> Discrete-Time Integrator/1, AND/1, Discrete-Time Integrator/2
  Compare To Constant/1 -> AND/2

== system AdmittanceScanPRBS/Renewable Plant/PV Plant/60 MWhr Battery Energy Storage/Variant Subsystem/Grid Forming VSM/GridFormingController/Current Limiting/CurrentLimitingMethod/currentSaturation/If Action Subsystem ==
  Is : Inport
  Isd : Inport  Port=2
  Isq : Inport  Port=3
  Action Port : ActionPort
  Constant : Constant  Value=maxSatCurrentLimit
  Divide : Product  Inputs=*/
  Product : Product
  Product1 : Product
  Idmax : Outport
  Iqmax : Outport  Port=2
  wires:
  Constant/1 -> Divide/1
  Is/1 -> Divide/2
  Divide/1 -> Product1/2, Product/1
  Isd/1 -> Product1/1
  Isq/1 -> Product/2
  Product1/1 -> Idmax/1
  Product/1 -> Iqmax/1

== system AdmittanceScanPRBS/Renewable Plant/PV Plant/60 MWhr Battery Energy Storage/Variant Subsystem/Grid Forming VSM/GridFormingController/Current Limiting/CurrentLimitingMethod/currentSaturation/If Action Subsystem1 ==
  Action Port : ActionPort
  Constant3 : Constant  Value=0
  Constant4 : Constant  Value=0
  Idmax : Outport
  Iqmax : Outport  Port=2
  wires:
  Constant4/1 -> Iqmax/1
  Constant3/1 -> Idmax/1

== system AdmittanceScanPRBS/Renewable Plant/PV Plant/60 MWhr Battery Energy Storage/Variant Subsystem/Grid Forming VSM/GridFormingController/Grid Voltage Reactive Power Support/Modifying Reactive Power Reference/Changing the Power Reference/ActivePowerReference ==
  note: Ensure Pref sign is maintained
  Id : Inport
  Vd : Inport  Port=2
  Pref : Inport  Port=3
  Abs1 : Abs  SaturateOnIntegerOverflow=off
  Abs2 : Abs  SaturateOnIntegerOverflow=off
  Min : MinMax  Inputs=2
  Product : Product
  Product2 : Product
  Saturation : Saturate  UpperLimit=1  LowerLimit=-1
  Sign : Signum
  PrefNew : Outport
  wires:
  Pref/1 -> Abs1/1, Sign/1
  Id/1 -> Product/1
  Sign/1 -> Product2/2
  Abs1/1 -> Min/2
  Product/1 -> Abs2/1
  Min/1 -> Product2/1
  Product2/1 -> Saturation/1
  Abs2/1 -> Min/1
  Vd/1 -> Product/2
  Saturation/1 -> PrefNew/1

== system AdmittanceScanPRBS/Renewable Plant/PV Plant/60 MWhr Battery Energy Storage/Variant Subsystem/Grid Forming VSM/GridFormingController/Grid Voltage Reactive Power Support/Modifying Reactive Power Reference/Changing the Power Reference/Estimate Id for Given Iq ==
  Iq : Inport
  Add Constant1 : Bias  Bias=1  SaturateOnIntegerOverflow=off
  Gain : Gain  Gain=-1
  Gain3 : Gain  Gain=0.9
  Sqrt : Sqrt
  Square : Math  Operator=square
  Id : Outport
  wires:
  Square/1 -> Gain/1
  Gain3/1 -> Id/1
  Gain/1 -> Add Constant1/1
  Sqrt/1 -> Gain3/1
  Add Constant1/1 -> Sqrt/1
  Iq/1 -> Square/1

== system AdmittanceScanPRBS/Renewable Plant/PV Plant/60 MWhr Battery Energy Storage/Variant Subsystem/Grid Forming VSM/GridFormingController/Grid Voltage Reactive Power Support/Modifying Reactive Power Reference/Changing the Power Reference/EstimateIqForReactivePower ==
  note: Computing minimum reactive current as per GC0137
  Vmin : Inport
  Vd : Inport  Port=2
  Vs : Inport  Port=3
  Abs : Abs  SaturateOnIntegerOverflow=off
  Add : Sum
  Add Constant : Bias  Bias=1  SaturateOnIntegerOverflow=off
  GC0137 line slope : Gain  Gain=-1.4578
  Low Voltage Support : Subsystem
  Saturation : Saturate  UpperLimit=1  LowerLimit=0
  Iq : Outport
  wires:
  Abs/1 -> GC0137 line slope/1
  GC0137 line slope/1 -> Add Constant/1
  Vs/1 -> Abs/1
  Add/1 -> Saturation/1
  Saturation/1 -> Iq/1
  Add Constant/1 -> Add/2
  Vmin/1 -> Low Voltage Support/1(Vin)
  Vd/1 -> Low Voltage Support/2(Vd)
  Low Voltage Support/1(Iqsupport) -> Add/1

== system AdmittanceScanPRBS/Renewable Plant/PV Plant/60 MWhr Battery Energy Storage/Variant Subsystem/Grid Forming VSM/GridFormingController/Grid Voltage Reactive Power Support/Modifying Reactive Power Reference/Changing the Power Reference/ReactivePowerReference ==
  Vd : Inport
  Iq : Inport  Port=2
  Compute Power : Product
  Constant : Constant  Value=0.3
  Gain2 : Gain  Gain=1.05
  Switch : Switch  Criteria=u2 > Threshold  Threshold=0.3  SaturateOnIntegerOverflow=off  InputSameDT=off
  QrefNew : Outport
  wires:
  Compute Power/1 -> QrefNew/1
  Gain2/1 -> Compute Power/2
  Constant/1 -> Switch/3
  Iq/1 -> Gain2/1
  Vd/1 -> Switch/2, Switch/1
  Switch/1 -> Compute Power/1

== system AdmittanceScanPRBS/Renewable Plant/PV Plant/60 MWhr Battery Energy Storage/Variant Subsystem/Grid Forming VSM/GridFormingController/Measurement/Frequency Measurement/Frequency Measurement/If Action Subsystem ==
  V : Inport
  Time : Inport  Port=2
  Action Port : ActionPort  ActionPortLabel=if(u1 > 0.9)
  Constant1 : Constant  Value=initialFrequency
  Delay : Delay  DelayLength=1
  Delay1 : Delay  DelayLength=1
  Frequency estimation : Subsystem  TreatAsAtomicUnit=on
  Hit Crossing : HitCross
  Switch : Switch  Criteria=u2 > Threshold  Threshold=1  SaturateOnIntegerOverflow=off  InputSameDT=off
  Freq : Outport
  wires:
  V/1 -> Delay/1, Frequency estimation/1(sk), Hit Crossing/1
  Delay1/1 -> Frequency estimation/4(k-1)
  Hit Crossing/1 -> Frequency estimation/Trigger
  Delay/1 -> Frequency estimation/2(sk-1)
  Time/1 -> Switch/2, Delay1/1, Frequency estimation/3(k)
  Frequency estimation/1(f) -> Switch/1
  Constant1/1 -> Switch/3
  Switch/1 -> Freq/1

== system AdmittanceScanPRBS/Renewable Plant/PV Plant/60 MWhr Battery Energy Storage/Variant Subsystem/Grid Forming VSM/GridFormingController/Measurement/Frequency Measurement/Frequency Measurement/If Action Subsystem1 ==
  Action Port : ActionPort  ActionPortLabel=else
  Constant1 : Constant  Value=initialFrequency
  Out1 : Outport
  wires:
  Constant1/1 -> Out1/1

== system AdmittanceScanPRBS/Renewable Plant/PV Plant/60 MWhr Battery Energy Storage/Variant Subsystem/Grid Forming VSM/GridFormingController/Measurement/Frequency Measurement/Frequency Measurement/Postive Sequence ==
  abc : Inport
  Complex to Real-Imag : ComplexToRealImag
  Demux : Demux  Outputs=3
  Symmetrical-Components Transform : eeTransforms/Symmetrical-Components Transform  PowerInvariant=off
      settings: LibrarySourceBlock=|
      | ee_sl_lib/Mathematical
      | Transforms/Symmetrical-Components
      | Transform
  Terminator : Terminator
  Terminator1 : Terminator
  Terminator2 : Terminator
  Transpose : Math  Operator=transpose
  posSeq : Outport
  wires:
  Transpose/1 -> Symmetrical-Components Transform/1
  Symmetrical-Components Transform/1 -> Demux/1
  Complex to Real-Imag/1 -> posSeq/1
  Demux/1 -> Complex to Real-Imag/1
  abc/1 -> Transpose/1
  Complex to Real-Imag/2 -> Terminator/1
  Demux/2 -> Terminator1/1
  Demux/3 -> Terminator2/1

== system AdmittanceScanPRBS/Renewable Plant/PV Plant/60 MWhr Battery Energy Storage/Variant Subsystem/Grid Forming VSM/GridFormingController/Power Control/ActivePowerControl/vsmControl/Damping Frequency ==
  fref : Inport
  ConstantFreqReference : Subsystem  VariantControl=constFreq
  WithFrequencyMeasurement : Subsystem  VariantControl=freqMeas
  fmeas : Outport

== system AdmittanceScanPRBS/Renewable Plant/PV Plant/60 MWhr Battery Energy Storage/Variant Subsystem/Grid Forming VSM/GridFormingController/Current Limiting/CurrentLimitingMethod/currentLimitAndVirtual/Current Saturation/Compare ==
  u : Inport
  Compare To Zero : simulink/Logic and Bit Operations/Compare To Zero  relop=<=  OutDataTypeStr=boolean
  Data Type Conversion : DataTypeConversion  SaturateOnIntegerOverflow=off  RndMeth=Floor
  Out1 : Outport
  wires:
  Compare To Zero/1 -> Data Type Conversion/1
  u/1 -> Compare To Zero/1
  Data Type Conversion/1 -> Out1/1

== system AdmittanceScanPRBS/Renewable Plant/PV Plant/60 MWhr Battery Energy Storage/Variant Subsystem/Grid Forming VSM/GridFormingController/Current Limiting/CurrentLimitingMethod/currentLimitAndVirtual/Current Saturation/If Action Subsystem ==
  Is : Inport
  Isd : Inport  Port=2
  Isq : Inport  Port=3
  maxI : Inport  Port=4
  Action Port : ActionPort
  Divide : Product  Inputs=*/
  Product : Product
  Product1 : Product
  Idmax : Outport
  Iqmax : Outport  Port=2
  wires:
  maxI/1 -> Divide/1
  Is/1 -> Divide/2
  Divide/1 -> Product1/2, Product/1
  Isd/1 -> Product1/1
  Isq/1 -> Product/2
  Product1/1 -> Idmax/1
  Product/1 -> Iqmax/1

== system AdmittanceScanPRBS/Renewable Plant/PV Plant/60 MWhr Battery Energy Storage/Variant Subsystem/Grid Forming VSM/GridFormingController/Current Limiting/CurrentLimitingMethod/currentLimitAndVirtual/Current Saturation/If Action Subsystem1 ==
  Action Port : ActionPort
  Constant3 : Constant  Value=0
  Constant4 : Constant  Value=0
  Idmax : Outport
  Iqmax : Outport  Port=2
  wires:
  Constant4/1 -> Iqmax/1
  Constant3/1 -> Idmax/1

== system AdmittanceScanPRBS/Renewable Plant/PV Plant/60 MWhr Battery Energy Storage/Variant Subsystem/Grid Forming VSM/GridFormingController/Grid Voltage Reactive Power Support/Modifying Reactive Power Reference/Changing the Power Reference/EstimateIqForReactivePower/Low Voltage Support ==
  Vin : Inport
  Vd : Inport  Port=2
  Gain4 : Gain  Gain=lowVoltageSupportGain
  Saturation1 : Saturate  UpperLimit=1  LowerLimit=-1
  Subtract : Sum  Inputs=+-
  Iqsupport : Outport
  wires:
  Subtract/1 -> Gain4/1
  Gain4/1 -> Saturation1/1
  Saturation1/1 -> Iqsupport/1
  Vin/1 -> Subtract/1
  Vd/1 -> Subtract/2

== system AdmittanceScanPRBS/Renewable Plant/PV Plant/60 MWhr Battery Energy Storage/Variant Subsystem/Grid Forming VSM/GridFormingController/Measurement/Frequency Measurement/Frequency Measurement/If Action Subsystem/Frequency estimation ==
  sk : Inport
  sk-1 : Inport  Port=2
  k : Inport  Port=3
  k-1 : Inport  Port=4
  Trigger : TriggerPort  VariantControl=(inherit)  InitialTriggerSignalState=positive
  Add1 : Sum  Inputs=+-  OutDataTypeStr=double  AccumDataTypeStr=double  RndMeth=Convergent
  Add2 : Sum
  Constant : Constant
  Delay : Delay  DelayLength=1
  Delay1 : Delay  DelayLength=1
  Divide : Product  Inputs=*/  RndMeth=Ceiling
  Gain : Gain  Gain=2  ParamDataTypeStr=double  RndMeth=Convergent
  Gain2 : Gain  Gain=0.5
  MATLAB Function : MATLAB Function  TreatAsAtomicUnit=on
  f : Outport
  wires:
  Add1/1 -> Gain/1
  Constant/1 -> Divide/1
  Gain/1 -> Divide/2
  MATLAB Function/1(x) -> Delay/1, Add1/1  "x1-y1/slope"
  Divide/1 -> Add2/1, Delay1/1
  Delay1/1 -> Add2/2
  Add2/1 -> Gain2/1
  Gain2/1 -> f/1
  Delay/1 -> Add1/2
  k/1 -> MATLAB Function/3(x1)
  k-1/1 -> MATLAB Function/4(x2)  "x1"
  sk/1 -> MATLAB Function/1(y1)
  sk-1/1 -> MATLAB Function/2(y2)

== system AdmittanceScanPRBS/Renewable Plant/PV Plant/60 MWhr Battery Energy Storage/Variant Subsystem/Grid Forming VSM/GridFormingController/Power Control/ActivePowerControl/vsmControl/Damping Frequency/ConstantFreqReference ==
  fref : Inport
  Constant1 : Constant
  Terminator : Terminator
  fmeas : Outport
  wires:
  Constant1/1 -> fmeas/1
  fref/1 -> Terminator/1

== system AdmittanceScanPRBS/Renewable Plant/PV Plant/60 MWhr Battery Energy Storage/Variant Subsystem/Grid Forming VSM/GridFormingController/Power Control/ActivePowerControl/vsmControl/Damping Frequency/WithFrequencyMeasurement ==
  fref : Inport
  fmeas : Outport
  wires:
  fref/1 -> fmeas/1

== matlab function AdmittanceScanPRBS/Renewable Plant/PV Plant/60 MWhr Battery Energy Storage/Variant Subsystem/Grid Forming VSM/GridFormingController/Measurement/Frequency Measurement/Frequency Measurement/If Action Subsystem/Frequency estimation/MATLAB Function ==
  data: y1 input; y2 input; x1 input; x output; x2 input
function x = fcn(y1,y2,x1,x2)
% Line equation between two points is y-y1=((y2-y1)/(x2-x1))*(x-x1). Here
% to to find the zero crossing instant substitute y = 0 and find x
slope = (y2-y1)/(x2-x1);
x = x1-y1/slope;

== stateflow chart AdmittanceScanPRBS/Renewable Plant/PV Plant/60 MWhr Battery Energy Storage/Variant Subsystem/Grid Forming VSM/GridFormingController/Current Limiting/CurrentLimitingMethod/currentLimitAndVirtual/CurrentLimitSelection ==
  state Mode1_VI_ON
    entry:
    noCurrentLimit  = 0;
    viCurrentLimit = 1;
    satCurrentLimit = 0;
    ismax= maxVICurrentLimit;
    exit:
    noCurrentLimit  = 0;
    viCurrentLimit = 1;
    satCurrentLimit = 0;
    ismax= maxVICurrentLimit;
  state Start_Mode
    entry:
    noCurrentLimit  = 1;
    viCurrentLimit = 0;
    satCurrentLimit = 0;
    ismax= maxSatCurrentLimit;
    exit:
    noCurrentLimit  = 1;
    viCurrentLimit = 0;
    satCurrentLimit = 0;
    ismax= maxSatCurrentLimit;
  state Mode2_CurrentSat_ON
    entry:
    noCurrentLimit  = 0;
    viCurrentLimit = 0;
    satCurrentLimit = 1;
    ismax= maxSatCurrentLimit;
    exit:
    noCurrentLimit  = 0;
    viCurrentLimit = 0;
    satCurrentLimit = 1;
    ismax= maxSatCurrentLimit;
  state Mode3_CurrentSat_ON
    entry:
    noCurrentLimit  = 0;
    viCurrentLimit = 0;
    satCurrentLimit = 1;
    ismax= maxVICurrentLimit;
    exit:
    noCurrentLimit  = 0;
    viCurrentLimit = 0;
    satCurrentLimit = 1;
    ismax= 0.97*maxVICurrentLimit;
  Start_Mode -> Mode1_VI_ON : [Is>1]
  (junction 28) -> Mode1_VI_ON : after(modeTransferTime, sec)[(Is<ismax) && (Is>1) ]
  Mode3_CurrentSat_ON -> (junction 28) [order 1]
  (default) -> Start_Mode
  Mode1_VI_ON -> Start_Mode [order 2] : [Is<1]
  Mode1_VI_ON -> Mode2_CurrentSat_ON [order 1] : after(1/powerFreq, sec)[(Is>=maxSatCurrentLimit)]
  (junction 26) -> Start_Mode
  Mode2_CurrentSat_ON -> Mode3_CurrentSat_ON : after(currentSatTime, sec)[satCurrentLimit>0]
  Mode3_CurrentSat_ON -> (junction 26) [order 2] : [Is<1]
  data: Is input; ismax output; noCurrentLimit output; viCurrentLimit output; satCurrentLimit output; maxSatCurrentLimit parameter; maxVICurrentLimit parameter; currentSatTime parameter; powerFreq parameter; modeTransferTime parameter
